simulink library "THB_set_mdot"  (Simulink 8.2)
settings: Solver=ode45  StartTime=0.0  StopTime=10.0  RelTol=1e-3
settings Model: Creator=lena.frank  LastModifiedBy=awohlfei

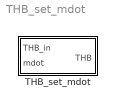
== system THB_set_mdot ==
  THB_set_mdot : Subsystem  InitFcn=load('THB.mat');  mask(set temperature in THB){}
      mask help: Set the mass flow rate in the thermo-hydraulic bus.
      mask Help: web(['file:///' fullfile(path_carnot('help'),'THB_set_mdot.html')],'-helpbrowser')

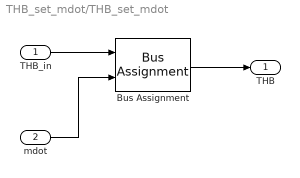
== system THB_set_mdot/THB_set_mdot ==
  THB_in : Inport
  mdot : Inport  Port=2
  Bus Assignment : BusAssignment  AssignedSignals=MassFlow
  THB : Outport
  wires:
  THB_in/1 -> Bus Assignment/1
  Bus Assignment/1 -> THB/1
  mdot/1 -> Bus Assignment/2
